simulink subsystem "PvtSubSys_VSM_SCM"  (R2020b)
settings: Solver=VariableStepAuto  StartTime=0.0  StopTime=10.0  RelTol=1e-3
undefined symbols (not defined in the file): P_Global_VehicleWidthMin_m, P_VSM_LDW_State_Param_LaneTime, P_VSM_LDW_State_Param_Speed, P_VSM_LKA_State_Param_Offset, P_VSM_LSMC_SampleTime
libraries: simulink x45
(part 2 of 3)

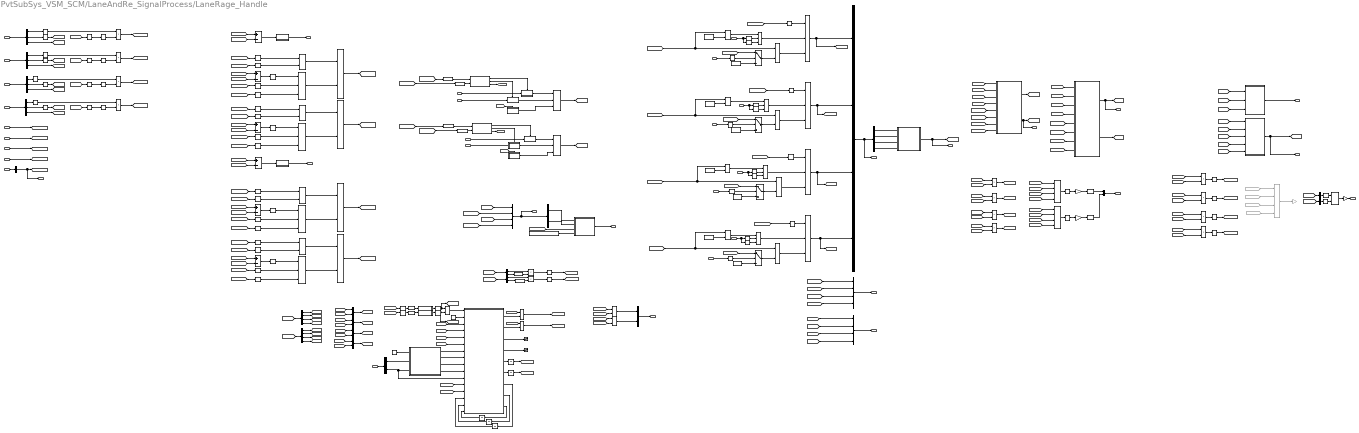
== system PvtSubSys_VSM_SCM/LaneAndRe_SignalProcess/LaneRage_Handle ==
  note: 该目标为相关侧有效
      | 车道线
  note: 注意：由于后期模块没有使用该
      | 输出（lane1）；所以去掉该输出
      | 接口；
      | 2020/10/12
  note: 目标车道线输出；
      | T_Valid为bool；
      | 其余皆为Single；
  note: 去掉了输出L信号；
      | 因为后面模块用不到；
  note: 车道线与车道边界之间差值（0.3m）；
  note: 存在数据类型问题：bool*double，需要求改
  Left_Lane : Inport
  Right_Lane : Inport  Port=2
  Left_Re : Inport  Port=3
  Right_Re : Inport  Port=4
  L_Lvalid : Inport  Port=5
  R_Lvalid : Inport  Port=6
  L_Revalid : Inport  Port=7
  R_Revalid : Inport  Port=8
  Center_lane : Inport  Port=9
  EVI : Inport  Port=10
  PilotSts : Inport  Port=11
  Abs{,1..13} (14 alike) : Abs
  Add{1..6} (6 alike) : Sum  Inputs=+-
  Atan : Trigonometry  Operator=atan
  Atan1 : Trigonometry  Operator=atan
  Bus Creator{,2,4,9} (4 alike) : BusCreator  Inputs=4
  Bus Creator{1,3,5..8} (6 alike) : BusCreator  Inputs=2
  Bus Selector : BusSelector  OutputSignals=Left_LaneValid,Right_LaneValid,Left_ReValid,Right_ReValid
  Bus Selector{1..4} (4 alike) : BusSelector  OutputSignals=A0,A1,A2
  Bus Selector10 : BusSelector  OutputSignals=A2
  Bus Selector11 : BusSelector  OutputSignals=A0,A1,A2,A3
  Bus Selector12 : BusSelector  OutputSignals=A0,A1,A2,A3
  Bus Selector13 : BusSelector  OutputSignals=Kap,VehicleSpd_ms
  Bus Selector5 : BusSelector  OutputSignals=A0,Valid
  Bus Selector6 : BusSelector  OutputSignals=A0,Valid
  Bus Selector7 : BusSelector  OutputSignals=Left_ValidLane,Right_ValidLane
  Bus Selector8 : BusSelector  OutputSignals=lane_Center
  Bus Selector9 : BusSelector  OutputSignals=A2
  CalcEgoVehMove1 : MATLAB Function  TreatAsAtomicUnit=on
  Compare To Constant{,23,37..38} (4 alike) : simulink/Logic and Bit Operations/Compare To Constant  relop=<  const=0.5  OutDataTypeStr=boolean
  Compare To Constant24 : simulink/Logic and Bit Operations/Compare To Constant  relop=>  const=4  OutDataTypeStr=boolean
  Compare To Constant25 : simulink/Logic and Bit Operations/Compare To Constant  relop=<  const=0  OutDataTypeStr=boolean
  Compare To Constant26 : simulink/Logic and Bit Operations/Compare To Constant  relop=>  const=0  OutDataTypeStr=boolean
  Compare To Constant34 : simulink/Logic and Bit Operations/Compare To Constant  relop=<  const=3.5  OutDataTypeStr=boolean
  Compare To Constant39 : simulink/Logic and Bit Operations/Compare To Constant  relop=>  const=0  OutDataTypeStr=boolean
  Compare To Constant40 : simulink/Logic and Bit Operations/Compare To Constant  relop=>  const=0  OutDataTypeStr=boolean
  Compare To Constant41 : simulink/Logic and Bit Operations/Compare To Constant  relop=>  const=0.2  OutDataTypeStr=boolean
  Compare To Constant42 : simulink/Logic and Bit Operations/Compare To Constant  relop=>  const=0.2  OutDataTypeStr=boolean
  Compare To Constant{47,49,51,53} (4 alike) : simulink/Logic and Bit Operations/Compare To Constant  relop===  const=2  OutDataTypeStr=boolean
  Compare To Constant{48,50,52,54} (4 alike) : simulink/Logic and Bit Operations/Compare To Constant  relop===  const=3  OutDataTypeStr=boolean
  Compare To Zero{,1,4..5,7..8,10..14,16..20,22..25,28..29} (22 alike) : simulink/Logic and Bit Operations/Compare To Zero  relop=>  OutDataTypeStr=boolean
  Compare To Zero2 : simulink/Logic and Bit Operations/Compare To Zero  relop=<  OutDataTypeStr=boolean
  Compare To Zero26 : simulink/Logic and Bit Operations/Compare To Zero  relop=<  OutDataTypeStr=boolean
  Constant1 : Constant  Value=[1,1]  OutDataTypeStr=uint8
  Constant{5,7,10,14} (4 alike) : Constant  Value=single(998)
  Constant{3,11,13,15} (4 alike) : Constant  Value=single(2.75)
  Constant12 : Constant  Value=0.02  OutDataTypeStr=single
  Constant9 : Constant  Value=P_VSM_LKA_State_Param_Offset
  Cos{,1..3} (4 alike) : Trigonometry  Operator=cos
  Data Type Conversion{,5..7,9..10} (6 alike) : DataTypeConversion
  Data Type Conversion2 : DataTypeConversion  OutDataTypeStr=double
  Data Type Conversion4 : DataTypeConversion  OutDataTypeStr=double
  Divide{,1..12,15} (14 alike) : Product  Inputs=**
  ELK_laneValid : MATLAB Function  TreatAsAtomicUnit=on
  From87 : From  Commented=on  GotoTag=Left_LaneA2
  From88 : From  Commented=on  GotoTag=Right_LaneA2
  From89 : From  Commented=on  GotoTag=Left_ReA2
  From90 : From  Commented=on  GotoTag=Right_ReA2
  Gain : Gain  Commented=on  Gain=2
  Gain1 : Gain  Gain=2
  Gain2 : Gain  Gain=57.3
  Gain3 : Gain  Gain=57.3
  If : If  NumInputs=2  ElseIfExpressions=u2>0
  If1 : If  NumInputs=2  ElseIfExpressions=u2>0
  L_Lvalid1 : InportShadow  Port=5
  L_Revalid1 : InportShadow  Port=7
  Left_Lane1 : InportShadow
  Left_Re1 : InportShadow  Port=3
  Logical Operator{,25,27,32..33,40..41} (7 alike) : Logic  Operator=OR  AllPortsSameDT=off  OutDataTypeStr=boolean
  Logical Operator{4..7,24,30..31,36} (8 alike) : Logic  Inputs=3  AllPortsSameDT=off  OutDataTypeStr=boolean
  Logical Operator{28..29,34..35,38..39} (6 alike) : Logic  AllPortsSameDT=off  OutDataTypeStr=boolean
  Logical Operator{44..47} (4 alike) : Logic  Operator=OR  Inputs=3  AllPortsSameDT=off  OutDataTypeStr=boolean
  MATLAB Function : MATLAB Function  TreatAsAtomicUnit=on
  MATLAB Function1 : MATLAB Function  TreatAsAtomicUnit=on
  MATLAB Function2 : MATLAB Function  TreatAsAtomicUnit=on
  Max : MinMax  Commented=on  Function=max  Inputs=4
  Max1 : MinMax  Function=max  Inputs=4
  Max2 : MinMax  Function=max  Inputs=4
  Max3 : MinMax  Function=max  Inputs=2
  Merge : Merge  Inputs=3
  Merge1 : Merge  Inputs=3
  PilotSts3 : InportShadow  Port=11
  PilotSts4 : InportShadow  Port=11
  PilotSts5 : InportShadow  Port=11
  R_Lvalid1 : InportShadow  Port=6
  R_Revalid1 : InportShadow  Port=8
  Relational Operator{1..4,9..10,13..14} (8 alike) : RelationalOperator  Operator=<  OutDataTypeStr=boolean  RndMeth=Nearest
  Right_Lane1 : InportShadow  Port=2
  Right_Re1 : InportShadow  Port=4
  SameTwoLaneCondition : MATLAB Function  TreatAsAtomicUnit=on
  SingleLaneCondition : MATLAB Function  TreatAsAtomicUnit=on
  Subsystem : Subsystem
  Subsystem4 : Subsystem  mask{Ts=P_VSM_LSMC_SampleTime, Max=10}
      mask prompts: Ts "Sample Time:"; Max "Max Limit:"
      mask Display:
      | Ts=get_param(gcb,'Ts');
      | Max=get_param(gcb,'Max');
      | disp(['Ts:' Ts '\n' 'Max:' Max ]);
  Subsystem6 : Subsystem  mask{Ts=P_VSM_LSMC_SampleTime, Max=10}
      mask prompts: Ts "Sample Time:"; Max "Max Limit:"
      mask Display:
      | Ts=get_param(gcb,'Ts');
      | Max=get_param(gcb,'Max');
      | disp(['Ts:' Ts '\n' 'Max:' Max ]);
  Switch Case Action Subsystem : Subsystem  TreatAsAtomicUnit=on
  Switch Case Action Subsystem1 : Subsystem  TreatAsAtomicUnit=on
  Switch Case Action Subsystem2 : Subsystem  TreatAsAtomicUnit=on
  Switch Case Action Subsystem3 : Subsystem  TreatAsAtomicUnit=on
  Switch Case Action Subsystem4 : Subsystem  TreatAsAtomicUnit=on
  Switch Case Action Subsystem5 : Subsystem  TreatAsAtomicUnit=on
  Switch{1,3,5,7} (4 alike) : Switch  Criteria=u2 > Threshold
  Terminator : Terminator
  Terminator2 : Terminator
  Tracker : MATLAB Function  TreatAsAtomicUnit=on
  TwoLaneCondition : MATLAB Function  TreatAsAtomicUnit=on
  Unit Delay{2..6} (5 alike) : UnitDelay  SampleTime=-1  HasFrameUpgradeWarning=on
  atan{,1..3} (4 alike) : Trigonometry  Operator=atan
  Left_LaneRe30 : Outport
  Right_LaneRe30 : Outport  Port=2
  LaneValid : Outport  Port=3
  HeadingAngle : Outport  Port=4
  LaneCurve : Outport  Port=5
  Valid_Lane : Outport  Port=6
  LaneChangeValid : Outport  Port=7
  Center_Lane : Outport  Port=8
  LDWLKAELK_LWidth : Outport  Port=9
  LSM_LCK_CLane : Outport  Port=10
  Related_Lane : Outport  Port=11
  LSS_RFMHandel_LaneA0 : Outport  Port=12
  Signal_Lane1 : Outport  Port=13
  Signal_Lane2 : Outport  Port=14
  Signal_Lane3 : Outport  Port=15
  LSS_RFM_LaneA1 : Outport  Port=16
  wires:
  Gain1/1 -> LaneCurve/1
  Max3/1 -> Gain1/1
  Bus Selector10/1 -> Abs12/1  "<A2>"
  Bus Selector9/1 -> Abs13/1  "<A2>"
  [Left_ValidLane] -> Bus Selector9/1
  [Right_ValidLane] -> Bus Selector10/1
  Constant9/1 -> Subsystem/4(Offset)
  [Center_Lane] -> Subsystem/3(CenterLane)
  Bus Selector8/1 -> LSM_LCK_CLane/1, [Center_Lane]  "<lane_Center>"
  Center_lane/1 -> Bus Selector8/1
  Bus Selector7/2 -> Subsystem/2(<Right_ValidLane>)  "<Right_ValidLane>"
  Bus Selector7/1 -> Subsystem/1(<Left_ValidLane>)  "<Left_ValidLane>"
  [Host_RRE] -> Bus Creator2/4  "Host_RRE"
  [Host_LRE] -> Bus Creator2/2  "Host_LRE"
  MATLAB Function2/1(y) -> Right_LaneRe30/1
  [Right_LaneOp_A0] -> Add3/2
  [Right_ReOp_A0] -> Add3/1
  Add3/1 -> MATLAB Function2/1(u)
  MATLAB Function1/1(y) -> Left_LaneRe30/1
  Compare To Zero29/1 -> Logical Operator31/3
  Compare To Zero28/1 -> Logical Operator31/2
  [Orginal_R_Lvalid] -> Compare To Zero28/1
  [Orginal_R_Revalid] -> Compare To Zero29/1
  [Orginal_R_Lvalid] -> Compare To Zero20/1
  Logical Operator31/1 -> Logical Operator32/2
  Compare To Zero20/1 -> Logical Operator35/1
  [Right_ReOp_A0] -> Add5/2
  [Right_LaneOp_A0] -> Add5/1
  Add5/1 -> Compare To Zero26/1
  Compare To Zero26/1 -> Logical Operator31/1
  [Orginal_R_Revalid] -> Compare To Constant23/1
  Compare To Constant23/1 -> Logical Operator35/2
  Logical Operator35/1 -> Logical Operator32/1
  Logical Operator32/1 -> [Host_RLane]
  Logical Operator34/1 -> Logical Operator33/1
  Compare To Zero22/1 -> Logical Operator34/2
  [Orginal_R_Revalid] -> Compare To Zero22/1
  Compare To Constant37/1 -> Logical Operator34/1
  [Orginal_R_Lvalid] -> Compare To Constant37/1
  Compare To Zero23/1 -> Logical Operator36/1
  Add6/1 -> Compare To Zero23/1
  [Right_LaneOp_A0] -> Add6/1
  [Right_ReOp_A0] -> Add6/2
  Logical Operator36/1 -> Logical Operator33/2
  [Orginal_R_Revalid] -> Compare To Zero25/1
  [Orginal_R_Lvalid] -> Compare To Zero24/1
  Compare To Zero24/1 -> Logical Operator36/2
  Compare To Zero25/1 -> Logical Operator36/3
  Logical Operator33/1 -> [Host_RRE]
  [Host_LRE] -> Data Type Conversion5/1
  [Host_LLane] -> Data Type Conversion/1
  Logical Operator27/1 -> [Host_LRE]
  Compare To Zero19/1 -> Logical Operator30/3
  Compare To Zero18/1 -> Logical Operator30/2
  [Orginal_L_Lvalid] -> Compare To Zero18/1
  [Orginal_L_Revalid] -> Compare To Zero19/1
  Logical Operator30/1 -> Logical Operator27/2
  [Left_ReOp_A0] -> Add4/2
  [Left_LaneOp_A0] -> Add4/1
  Add4/1 -> Compare To Zero17/1
  Compare To Zero17/1 -> Logical Operator30/1
  [Orginal_L_Lvalid] -> Compare To Constant/1
  Compare To Constant/1 -> Logical Operator28/1
  [Orginal_L_Revalid] -> Compare To Zero16/1
  Compare To Zero16/1 -> Logical Operator28/2
  Logical Operator28/1 -> Logical Operator27/1
  Logical Operator25/1 -> [Host_LLane]
  Logical Operator29/1 -> Logical Operator25/1
  Compare To Constant38/1 -> Logical Operator29/2
  [Orginal_L_Revalid] -> Compare To Constant38/1
  [Left_LaneOp_A0] -> Add2/2
  [Left_ReOp_A0] -> Add2/1
  Compare To Zero2/1 -> Logical Operator24/1
  Add1/1 -> Compare To Zero2/1
  [Left_LaneOp_A0] -> Add1/1
  [Left_ReOp_A0] -> Add1/2
  Compare To Zero12/1 -> Logical Operator29/1
  Logical Operator24/1 -> Logical Operator25/2
  [Orginal_L_Lvalid] -> Compare To Zero12/1
  [Orginal_L_Revalid] -> Compare To Zero5/1
  [Orginal_L_Lvalid] -> Compare To Zero4/1
  Compare To Zero4/1 -> Logical Operator24/2
  Compare To Zero5/1 -> Logical Operator24/3
  Add2/1 -> MATLAB Function1/1(u)
  Bus Creator3/1 -> LaneChangeValid/1
  Compare To Constant26/1 -> [RightChange_old]  "VSM_RightChange_old"
  Compare To Constant25/1 -> [LeftChange_old]  "VSM_LeftChange_old"
  Switch Case Action Subsystem5/1(Out1) -> Merge1/3
  [Right_else] -> Switch Case Action Subsystem5/Action
  Switch Case Action Subsystem4/1(Out1) -> Merge/3
  [Left_else] -> Switch Case Action Subsystem4/Action
  Divide12/1 -> Compare To Constant26/1
  Divide11/1 -> Compare To Constant25/1
  Bus Selector6/2 -> Data Type Conversion9/1  "<Valid>"
  Bus Selector6/1 -> Divide12/1  "<A0>"
  Bus Selector5/2 -> Data Type Conversion10/1  "<Valid>"
  Bus Selector5/1 -> Divide11/1  "<A0>"
  [Right_ValidLane] -> Bus Selector6/1  "Right_ValidLane"
  [Left_ValidLane] -> Bus Selector5/1  "Left_ValidLane"
  Bus Creator2/1 -> Valid_Lane/1, Bus Selector7/1
  [Right_ValidLane] -> Bus Creator2/3  "Right_ValidLane"
  [Left_ValidLane] -> Bus Creator2/1  "Left_ValidLane"
  Data Type Conversion7/1 -> If1/2
  Data Type Conversion6/1 -> If1/1
  Data Type Conversion5/1 -> If/2
  Data Type Conversion/1 -> If/1
  Merge1/1 -> [Right_ValidLane]
  Merge/1 -> [Left_ValidLane]
  If1/3 -> [Right_else]
  Switch Case Action Subsystem3/1(Out1) -> Merge1/2
  Switch Case Action Subsystem2/1(Out1) -> Merge1/1
  If1/2 -> Switch Case Action Subsystem3/Action
  If1/1 -> Switch Case Action Subsystem2/Action
  Right_Re1/1 -> Switch Case Action Subsystem3/1(In1)  "Right_Re"
  Right_Lane1/1 -> Switch Case Action Subsystem2/1(In1)  "Right_Lane"
  Switch Case Action Subsystem1/1(Out1) -> Merge/2
  Switch Case Action Subsystem/1(Out1) -> Merge/1
  If/3 -> [Left_else]
  [Host_RRE] -> Data Type Conversion7/1
  [Host_RLane] -> Data Type Conversion6/1
  If/2 -> Switch Case Action Subsystem1/Action
  Left_Re1/1 -> Switch Case Action Subsystem1/1(In1)  "Left_Re"
  If/1 -> Switch Case Action Subsystem/Action
  Left_Lane1/1 -> Switch Case Action Subsystem/1(In1)  "Left_Lane"
  From89/1 -> Max/3
  From90/1 -> Max/4
  From88/1 -> Max/2
  From87/1 -> Max/1
  Abs11/1 -> [Right_ReA2]
  Abs10/1 -> [Left_ReA2]
  Abs9/1 -> [Right_LaneA2]
  Abs8/1 -> [Left_LaneA2]
  Divide10/1 -> Abs11/1
  Divide9/1 -> Abs10/1
  [Right_Re_A2] -> Divide10/2
  [Right_ReValid] -> Divide10/1
  [Left_Re_A2] -> Divide9/2
  [Left_ReValid] -> Divide9/1
  [Right_Lane_A2] -> Divide8/2
  [Right_LaneValid] -> Divide8/1
  Bus Selector4/3 -> [Right_Re_A2]  "<A2>"
  Bus Selector3/3 -> [Left_Re_A2]  "<A2>"
  Bus Selector2/3 -> [Right_Lane_A2]  "<A2>"
  Bus Selector1/3 -> [Left_Lane_A2]  "<A2>"
  Bus Selector3/2 -> Abs5/1  "<A1>"
  [Left_LaneValid] -> Divide15/1
  Divide8/1 -> Abs9/1
  [Left_Lane_A2] -> Divide15/2
  Max/1 -> Gain/1
  Divide15/1 -> Abs8/1
  Bus Creator1/1 -> HeadingAngle/1
  [Right_ReA1] -> Max2/4
  [Left_ReA1] -> Max2/3
  [Right_LaneA1] -> Max2/2
  [Left_LaneA1] -> Max2/1
  [Right_ReA1] -> Max1/4
  [Left_ReA1] -> Max1/3
  [Right_LaneA1] -> Max1/2
  [Left_LaneA1] -> Max1/1
  Divide7/1 -> [Right_ReA1]
  Divide6/1 -> [Left_ReA1]
  Divide5/1 -> [Right_LaneA1]
  Divide4/1 -> [Left_LaneA1]
  Compare To Constant24/1 -> Bus Creator1/2  "HeadingAngle_Out"
  Atan1/1 -> Gain3/1
  Max2/1 -> Atan1/1
  [Right_ReValid] -> Divide7/2
  [Right_Re_A1] -> Divide7/1
  [Left_ReValid] -> Divide6/2
  [Left_Re_A1] -> Divide6/1
  [Right_LaneValid] -> Divide5/2
  [Right_Lane_A1] -> Divide5/1
  [Left_LaneValid] -> Divide4/2
  [Left_Lane_A1] -> Divide4/1
  Max1/1 -> Atan/1
  Atan/1 -> Gain2/1
  Compare To Constant34/1 -> Bus Creator1/1  "HeadingAngle_In"
  Abs7/1 -> [Right_Re_A1]
  Abs5/1 -> [Left_Re_A1]
  Abs3/1 -> [Right_Lane_A1]
  Abs1/1 -> [Left_Lane_A1]
  [Right_ReOp_A0] -> SameTwoLaneCondition/8(reright)
  [Left_ReOp_A0] -> SameTwoLaneCondition/7(releft)
  [Right_LaneOp_A0] -> SameTwoLaneCondition/6(laneright)
  [Left_LaneOp_A0] -> SameTwoLaneCondition/5(laneleft)
  Divide3/1 -> [Right_ReOp_A0]
  Divide2/1 -> [Left_ReOp_A0]
  Divide1/1 -> [Right_LaneOp_A0]
  Divide/1 -> [Left_LaneOp_A0]
  Cos3/1 -> Divide3/2
  atan3/1 -> Cos3/1
  [Right_Re_A1] -> atan3/1
  Abs6/1 -> Divide3/1
  Cos2/1 -> Divide2/2
  atan2/1 -> Cos2/1
  [Left_Re_A1] -> atan2/1
  Abs4/1 -> Divide2/1
  atan1/1 -> Cos1/1
  Cos1/1 -> Divide1/2
  [Right_Lane_A1] -> atan1/1
  Abs2/1 -> Divide1/1
  Abs/1 -> Divide/1
  Cos/1 -> Divide/2
  atan/1 -> Cos/1
  [Left_Lane_A1] -> atan/1
  Bus Selector4/2 -> Abs7/1  "<A1>"
  Bus Selector4/1 -> Abs6/1  "<A0>"
  Bus Selector3/1 -> Abs4/1  "<A0>"
  Bus Selector2/1 -> Abs2/1  "<A0>"
  Bus Selector2/2 -> Abs3/1  "<A1>"
  Bus Selector1/2 -> Abs1/1  "<A1>"
  Bus Selector1/1 -> Abs/1  "<A0>"
  Right_Re/1 -> Bus Selector4/1  "Right_Re"
  Left_Re/1 -> Bus Selector3/1  "Left_Re"
  Right_Lane/1 -> Bus Selector2/1  "Right_Lane"
  Left_Lane/1 -> Bus Selector1/1  "Left_Lane"
  MATLAB Function/1(L) -> LDWLKAELK_LWidth/1, [L]  "VSM_ELK_LWidth"
  [lane1] -> MATLAB Function/1(lane1)
  [lane3] -> MATLAB Function/3(lane3)
  [lane2] -> MATLAB Function/2(lane2)
  [L2] -> MATLAB Function/5(L2)
  [L1] -> MATLAB Function/4(L1)
  [lane3] -> ELK_laneValid/3(lane3)
  SameTwoLaneCondition/1(L1) -> [L1]
  Logical Operator4/1 -> [Left_ReValid], Bus Creator/3  "Left_ReValid"
  Logical Operator7/1 -> [Right_ReValid], Bus Creator/4  "Right_ReValid"
  [Left_ReValid] -> TwoLaneCondition/3(releft_valid)
  [Right_ReValid] -> TwoLaneCondition/4(reright_valid)
  [Left_LaneOp_A0] -> TwoLaneCondition/5(laneleft)  "Left_Lane"
  [Right_LaneOp_A0] -> TwoLaneCondition/6(laneright)  "Right_Lane"
  [Left_ReOp_A0] -> TwoLaneCondition/7(releft)  "Left_Re"
  [Right_ReOp_A0] -> TwoLaneCondition/8(reright)  "Right_Re"
  SingleLaneCondition/1(lane) -> Signal_Lane1/1, [lane1]  "lane1"
  SameTwoLaneCondition/2(lane) -> Signal_Lane2/1, [lane2]
  TwoLaneCondition/1(lane) -> Signal_Lane3/1, [lane3]
  Bus Creator/1 -> Related_Lane/1, Bus Selector/1
  [lane1] -> ELK_laneValid/1(lane1)
  [lane2] -> ELK_laneValid/2(lane2)
  ELK_laneValid/1(y) -> LaneValid/1
  TwoLaneCondition/2(L2) -> [L2]
  Logical Operator6/1 -> [Right_LaneValid], Bus Creator/2  "Right_LaneValid"
  Logical Operator5/1 -> [Left_LaneValid], Bus Creator/1  "Left_LaneValid"
  Compare To Zero/1 -> Logical Operator5/1
  Relational Operator9/1 -> Logical Operator5/3
  [Left_LaneOp_A0] -> Relational Operator1/1, Relational Operator9/1  "Left_Lane"
  [Left_LaneValid] -> TwoLaneCondition/1(laneleft_valid)
  [Right_LaneValid] -> TwoLaneCondition/2(laneright_valid)
  [Left_ReOp_A0] -> Switch1/1  "Left_Re"
  Switch1/1 -> Relational Operator9/2
  Constant14/1 -> Switch1/3
  Compare To Zero7/1 -> Switch1/2
  L_Revalid1/1 -> Compare To Zero7/1
  R_Revalid1/1 -> Compare To Zero10/1
  Compare To Zero10/1 -> Switch3/2
  Constant5/1 -> Switch3/3
  Switch3/1 -> Relational Operator13/2
  [Right_ReOp_A0] -> Switch3/1  "Right_Re"
  [Right_LaneOp_A0] -> Relational Operator2/1, Relational Operator13/1  "Right_Lane"
  Relational Operator13/1 -> Logical Operator6/3
  Compare To Zero8/1 -> Logical Operator6/1
  Compare To Zero11/1 -> Logical Operator4/1
  Relational Operator10/1 -> Logical Operator4/3
  [Left_ReOp_A0] -> Relational Operator3/1, Relational Operator10/1  "Left_Re"
  [Left_LaneOp_A0] -> Switch5/1  "Left_Lane"
  Switch5/1 -> Relational Operator10/2
  Constant10/1 -> Switch5/3
  Compare To Zero1/1 -> Switch5/2
  L_Lvalid1/1 -> Compare To Zero1/1
  R_Lvalid1/1 -> Compare To Zero13/1
  Compare To Zero13/1 -> Switch7/2
  Constant7/1 -> Switch7/3
  Switch7/1 -> Relational Operator14/2
  [Right_LaneOp_A0] -> Switch7/1  "Right_Lane"
  [Right_ReOp_A0] -> Relational Operator4/1, Relational Operator14/1  "Right_Re"
  Relational Operator14/1 -> Logical Operator7/3
  Compare To Zero14/1 -> Logical Operator7/1
  Constant13/1 -> Relational Operator1/2
  Constant3/1 -> Relational Operator2/2
  Constant11/1 -> Relational Operator3/2
  Constant15/1 -> Relational Operator4/2
  Bus Selector/1 -> SingleLaneCondition/1(laneleft_valid)  "<Left_LaneValid>"
  Bus Selector/2 -> SingleLaneCondition/2(laneright_valid)  "<Right_LaneValid>"
  Bus Selector/3 -> SingleLaneCondition/3(releft_valid)  "<Left_ReValid>"
  Bus Selector/4 -> SingleLaneCondition/4(reright_valid)  "<Right_ReValid>"
  [Left_LaneValid] -> SameTwoLaneCondition/1(laneleft_valid)
  [Right_LaneValid] -> SameTwoLaneCondition/2(laneright_valid)
  [Left_ReValid] -> SameTwoLaneCondition/3(releft_valid)
  [Right_ReValid] -> SameTwoLaneCondition/4(reright_valid)
  L_Lvalid/1 -> [Orginal_L_Lvalid]
  R_Lvalid/1 -> [Orginal_R_Lvalid]
  L_Revalid/1 -> [Orginal_L_Revalid]
  R_Revalid/1 -> [Orginal_R_Revalid]
  [Orginal_L_Lvalid] -> Compare To Zero/1
  [Orginal_R_Lvalid] -> Compare To Zero8/1
  [Orginal_L_Revalid] -> Compare To Zero11/1
  [Orginal_R_Revalid] -> Compare To Zero14/1
  Subsystem/1(Out1) -> Center_Lane/1
  Data Type Conversion9/1 -> Divide12/2
  Data Type Conversion10/1 -> Divide11/2
  Gain2/1 -> Compare To Constant34/1
  Gain3/1 -> Compare To Constant24/1
  Abs12/1 -> Max3/2
  Abs13/1 -> Max3/1
  [Right_LaneValid] -> Compare To Constant40/1
  [A1] -> Tracker/4(A1)
  Bus Selector11/3 -> [LA2]  "<A2>"
  Bus Creator8/1 -> [A3]
  Logical Operator41/1 -> Bus Creator3/2  "RightChange"
  [RightChange_old] -> Logical Operator41/1
  Tracker/7(pre_A1_1) -> Unit Delay6/1
  Bus Creator5/1 -> [A0]
  Logical Operator40/1 -> Bus Creator3/1  "LeftChange"
  [LValid] -> Logical Operator38/1
  [RightChange_new] -> Logical Operator41/2
  Data Type Conversion2/1 -> Subsystem4/1(In1)
  Compare To Constant41/1 -> [RValid], Logical Operator/2
  Tracker/3(error_right) -> Terminator2/1  "VSM_ERROR_RIGHT"
  [LeftChange_new] -> Logical Operator40/2
  Compare To Constant39/1 -> Data Type Conversion4/1
  [RA2] -> Bus Creator7/1
  [LeftChange_old] -> Logical Operator40/1
  Bus Selector12/2 -> [RA1]  "<A1>"
  Bus Selector12/1 -> [RA0]  "<A0>"
  [pre_A1_2K1] -> Tracker/12(pre_A1_2K1)
  Compare To Constant42/1 -> [LValid], Logical Operator/1
  Bus Selector11/2 -> [LA1]  "<A1>"
  Bus Selector11/1 -> [LA0]  "<A0>"
  [RValid] -> Logical Operator39/1
  Subsystem4/1(Out1) -> Compare To Constant41/1
  Tracker/2(RightOffset_b) -> Logical Operator39/2
  CalcEgoVehMove1/4(SinOfPsi) -> Tracker/10(SinOfPsi)
  Unit Delay2/1 -> [pre_A1_2K1]
  [pre_A0_2K1] -> Tracker/13(pre_A0_2K1)
  Tracker/1(LeftOffset_b) -> Logical Operator38/2
  Logical Operator38/1 -> [LeftChange_new]  "VSM_LeftChange_new"
  Unit Delay3/1 -> [pre_A0_2K1]
  Bus Creator6/1 -> [A1]
  Tracker/5(pre_A1_2) -> Unit Delay2/1
  Logical Operator39/1 -> [RightChange_new]  "VSM_RightChange_new"
  Bus Selector13/2 -> CalcEgoVehMove1/3(Vego), Tracker/11(vRef)  "<VehicleSpd_ms>"
  CalcEgoVehMove1/3(CosOfPsi) -> Tracker/9(CosOfPsi)
  Unit Delay6/1 -> Tracker/14(pre_A1_1K1)
  Tracker/8(pre_A0_1) -> Unit Delay5/1
  Unit Delay4/1 -> Tracker/16(pre_LineConfK1)
  Bus Selector13/1 -> CalcEgoVehMove1/2(Kap)  "<Kap>"
  [Left_ValidLane] -> Bus Selector11/1
  [Left_LaneValid] -> Compare To Constant39/1
  Data Type Conversion4/1 -> Subsystem6/1(In1)
  EVI/1 -> Bus Selector13/1
  Subsystem6/1(Out1) -> Compare To Constant42/1
  Tracker/9(pre_LineConf) -> Unit Delay4/1
  Compare To Constant40/1 -> Data Type Conversion2/1
  [LA2] -> Bus Creator7/2
  Constant1/1 -> Tracker/2(LineConf)
  [LA3] -> Bus Creator8/2
  Constant12/1 -> CalcEgoVehMove1/1(tCycle)
  [A0] -> Tracker/3(A0)
  [A2] -> Tracker/5(A2)
  [RA3] -> Bus Creator8/1
  Unit Delay5/1 -> Tracker/15(pre_A0_1K1)
  [A3] -> Tracker/6(A3)
  Bus Creator7/1 -> [A2]
  [LA1] -> Bus Creator6/2
  Bus Selector11/4 -> [LA3]  "<A3>"
  [RA1] -> Bus Creator6/1
  Logical Operator/1 -> Tracker/1(LineUpdate)
  Bus Selector12/4 -> [RA3]  "<A3>"
  CalcEgoVehMove1/1(dDeltaX) -> Tracker/7(dDeltaX)
  [Right_ValidLane] -> Bus Selector12/1
  Tracker/4(error_left) -> Terminator/1  "VSM_ERROR_LEFT"
  [LA0] -> Bus Creator5/2
  Tracker/6(pre_A0_2) -> Unit Delay3/1
  [RA0] -> Bus Creator5/1
  CalcEgoVehMove1/2(dDeltaY) -> Tracker/8(dDeltaY)
  Bus Selector12/3 -> [RA2]  "<A2>"
  Compare To Constant47/1 -> Logical Operator44/2
  Compare To Constant48/1 -> Logical Operator44/3
  PilotSts/1 -> Compare To Constant47/1, Compare To Constant48/1
  Relational Operator1/1 -> Logical Operator44/1
  Logical Operator44/1 -> Logical Operator5/2
  PilotSts3/1 -> Compare To Constant50/1, Compare To Constant49/1
  Compare To Constant50/1 -> Logical Operator45/3
  Compare To Constant49/1 -> Logical Operator45/2
  Relational Operator2/1 -> Logical Operator45/1
  Logical Operator45/1 -> Logical Operator6/2
  Compare To Constant51/1 -> Logical Operator46/2
  Compare To Constant52/1 -> Logical Operator46/3
  PilotSts4/1 -> Compare To Constant51/1, Compare To Constant52/1
  Relational Operator3/1 -> Logical Operator46/1
  Logical Operator46/1 -> Logical Operator4/2
  PilotSts5/1 -> Compare To Constant54/1, Compare To Constant53/1
  Compare To Constant54/1 -> Logical Operator47/3
  Compare To Constant53/1 -> Logical Operator47/2
  Relational Operator4/1 -> Logical Operator47/1
  Logical Operator47/1 -> Logical Operator7/2
  [Left_LaneOp_A0] -> Bus Creator4/1  "Left_LaneOp_A0"
  [Right_LaneOp_A0] -> Bus Creator4/2  "Right_LaneOp_A0"
  [Left_ReOp_A0] -> Bus Creator4/3  "Left_ReOp_A0"
  [Right_ReOp_A0] -> Bus Creator4/4  "Right_ReOp_A0"
  Bus Creator4/1 -> LSS_RFMHandel_LaneA0/1
  [Left_Lane_A1] -> Bus Creator9/1  "Left_Lane_A1"
  [Right_Lane_A1] -> Bus Creator9/2  "Right_Lane_A1"
  [Left_Re_A1] -> Bus Creator9/3  "Left_Re_A1"
  [Right_Re_A1] -> Bus Creator9/4  "Right_Re_A1"
  Bus Creator9/1 -> LSS_RFM_LaneA1/1

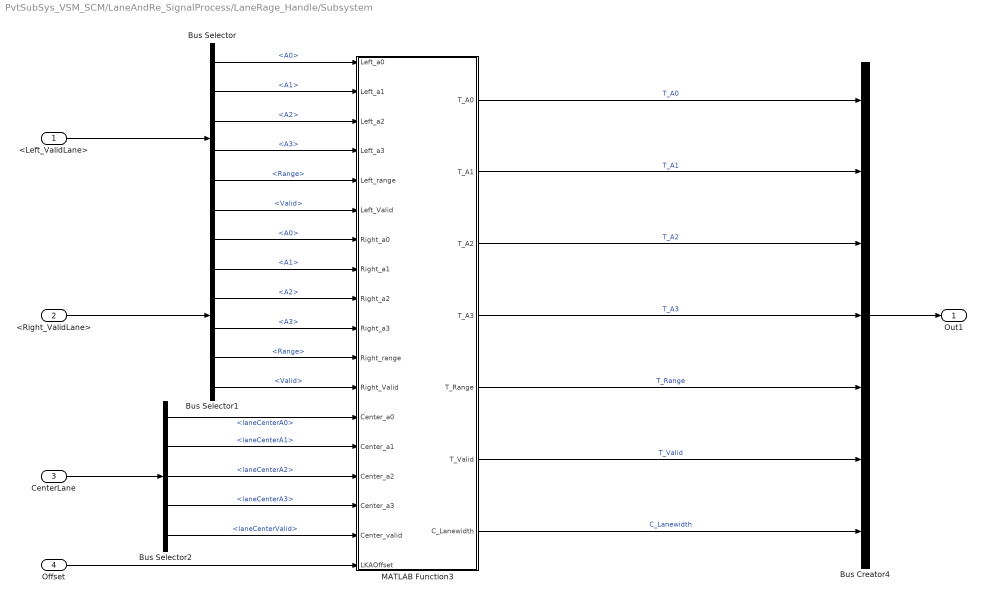
== system PvtSubSys_VSM_SCM/LaneAndRe_SignalProcess/LaneRage_Handle/Subsystem ==
  <Left_ValidLane> : Inport
  <Right_ValidLane> : Inport  Port=2
  CenterLane : Inport  Port=3
  Offset : Inport  Port=4
  Bus Creator4 : BusCreator  Inputs=7
  Bus Selector : BusSelector  OutputSignals=A0,A1,A2,A3,Range,Valid
  Bus Selector1 : BusSelector  OutputSignals=A0,A1,A2,A3,Range,Valid
  Bus Selector2 : BusSelector  OutputSignals=laneCenterA0,laneCenterA1,laneCenterA2,laneCenterA3,laneCenterValid
  MATLAB Function3 : MATLAB Function  TreatAsAtomicUnit=on
  Out1 : Outport
  wires:
  MATLAB Function3/1(T_A0) -> Bus Creator4/1  "T_A0"
  MATLAB Function3/5(T_Range) -> Bus Creator4/5  "T_Range"
  MATLAB Function3/3(T_A2) -> Bus Creator4/3  "T_A2"
  MATLAB Function3/2(T_A1) -> Bus Creator4/2  "T_A1"
  MATLAB Function3/7(C_Lanewidth) -> Bus Creator4/7  "C_Lanewidth"
  MATLAB Function3/4(T_A3) -> Bus Creator4/4  "T_A3"
  MATLAB Function3/6(T_Valid) -> Bus Creator4/6  "T_Valid"
  Offset/1 -> MATLAB Function3/18(LKAOffset)
  Bus Creator4/1 -> Out1/1
  <Left_ValidLane>/1 -> Bus Selector/1
  <Right_ValidLane>/1 -> Bus Selector1/1
  CenterLane/1 -> Bus Selector2/1
  Bus Selector/1 -> MATLAB Function3/1(Left_a0)  "<A0>"
  Bus Selector/2 -> MATLAB Function3/2(Left_a1)  "<A1>"
  Bus Selector/3 -> MATLAB Function3/3(Left_a2)  "<A2>"
  Bus Selector/4 -> MATLAB Function3/4(Left_a3)  "<A3>"
  Bus Selector/5 -> MATLAB Function3/5(Left_range)  "<Range>"
  Bus Selector/6 -> MATLAB Function3/6(Left_Valid)  "<Valid>"
  Bus Selector1/1 -> MATLAB Function3/7(Right_a0)  "<A0>"
  Bus Selector1/2 -> MATLAB Function3/8(Right_a1)  "<A1>"
  Bus Selector1/3 -> MATLAB Function3/9(Right_a2)  "<A2>"
  Bus Selector1/4 -> MATLAB Function3/10(Right_a3)  "<A3>"
  Bus Selector1/5 -> MATLAB Function3/11(Right_range)  "<Range>"
  Bus Selector1/6 -> MATLAB Function3/12(Right_Valid)  "<Valid>"
  Bus Selector2/1 -> MATLAB Function3/13(Center_a0)  "<laneCenterA0>"
  Bus Selector2/2 -> MATLAB Function3/14(Center_a1)  "<laneCenterA1>"
  Bus Selector2/3 -> MATLAB Function3/15(Center_a2)  "<laneCenterA2>"
  Bus Selector2/4 -> MATLAB Function3/16(Center_a3)  "<laneCenterA3>"
  Bus Selector2/5 -> MATLAB Function3/17(Center_valid)  "<laneCenterValid>"

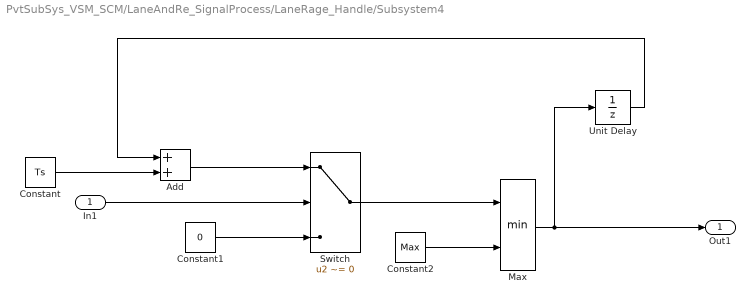
== system PvtSubSys_VSM_SCM/LaneAndRe_SignalProcess/LaneRage_Handle/Subsystem4 ==
  In1 : Inport
  Add : Sum
  Constant : Constant  Value=Ts
  Constant1 : Constant  Value=0
  Constant2 : Constant  Value=Max
  Max : MinMax  Inputs=2
  Switch : Switch  Criteria=u2 ~= 0
  Unit Delay : UnitDelay  SampleTime=-1  HasFrameUpgradeWarning=on
  Out1 : Outport
  wires:
  Switch/1 -> Max/1
  Constant2/1 -> Max/2
  Max/1 -> Out1/1, Unit Delay/1
  Add/1 -> Switch/1
  Constant1/1 -> Switch/3
  Constant/1 -> Add/2
  In1/1 -> Switch/2
  Unit Delay/1 -> Add/1

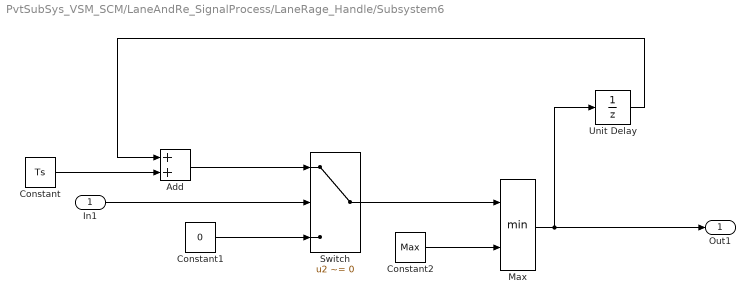
== system PvtSubSys_VSM_SCM/LaneAndRe_SignalProcess/LaneRage_Handle/Subsystem6 ==
  In1 : Inport
  Add : Sum
  Constant : Constant  Value=Ts
  Constant1 : Constant  Value=0
  Constant2 : Constant  Value=Max
  Max : MinMax  Inputs=2
  Switch : Switch  Criteria=u2 ~= 0
  Unit Delay : UnitDelay  SampleTime=-1  HasFrameUpgradeWarning=on
  Out1 : Outport
  wires:
  Unit Delay/1 -> Add/1
  In1/1 -> Switch/2
  Constant/1 -> Add/2
  Constant1/1 -> Switch/3
  Add/1 -> Switch/1
  Max/1 -> Unit Delay/1, Out1/1
  Constant2/1 -> Max/2
  Switch/1 -> Max/1

== system PvtSubSys_VSM_SCM/LaneAndRe_SignalProcess/LaneRage_Handle/Switch Case Action Subsystem ==
  In1 : Inport
  Action Port : ActionPort
  Bus Creator : BusCreator  Inputs=7
  Bus Selector : BusSelector  OutputSignals=A0,A1,A2,A3,Range,Valid,Left_Type
  Out1 : Outport
  wires:
  Bus Selector/7 -> Bus Creator/7  "<Left_Type>"
  Bus Creator/1 -> Out1/1
  Bus Selector/5 -> Bus Creator/5  "<Range>"
  Bus Selector/1 -> Bus Creator/1  "<A0>"
  Bus Selector/6 -> Bus Creator/6  "<Valid>"
  Bus Selector/2 -> Bus Creator/2  "<A1>"
  Bus Selector/4 -> Bus Creator/4  "<A3>"
  Bus Selector/3 -> Bus Creator/3  "<A2>"
  In1/1 -> Bus Selector/1

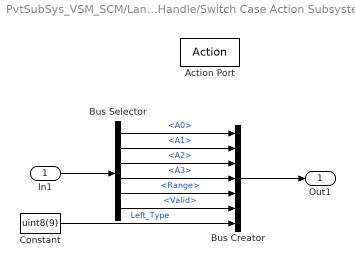
== system PvtSubSys_VSM_SCM/LaneAndRe_SignalProcess/LaneRage_Handle/Switch Case Action Subsystem1 ==
  In1 : Inport
  Action Port : ActionPort
  Bus Creator : BusCreator  Inputs=7
  Bus Selector : BusSelector  OutputSignals=A0,A1,A2,A3,Range,Valid
  Constant : Constant  Value=uint8(9)
  Out1 : Outport
  wires:
  Constant/1 -> Bus Creator/7  "Left_Type"
  In1/1 -> Bus Selector/1
  Bus Selector/3 -> Bus Creator/3  "<A2>"
  Bus Selector/4 -> Bus Creator/4  "<A3>"
  Bus Selector/2 -> Bus Creator/2  "<A1>"
  Bus Selector/6 -> Bus Creator/6  "<Valid>"
  Bus Selector/1 -> Bus Creator/1  "<A0>"
  Bus Selector/5 -> Bus Creator/5  "<Range>"
  Bus Creator/1 -> Out1/1

== system PvtSubSys_VSM_SCM/LaneAndRe_SignalProcess/LaneRage_Handle/Switch Case Action Subsystem2 ==
  In1 : Inport
  Action Port : ActionPort
  Bus Creator : BusCreator  Inputs=7
  Bus Selector : BusSelector  OutputSignals=A0,A1,A2,A3,Range,Valid,Right_Type
  Out1 : Outport
  wires:
  Bus Selector/7 -> Bus Creator/7  "<Right_Type>"
  Bus Creator/1 -> Out1/1
  Bus Selector/5 -> Bus Creator/5  "<Range>"
  Bus Selector/1 -> Bus Creator/1  "<A0>"
  Bus Selector/6 -> Bus Creator/6  "<Valid>"
  Bus Selector/2 -> Bus Creator/2  "<A1>"
  Bus Selector/4 -> Bus Creator/4  "<A3>"
  Bus Selector/3 -> Bus Creator/3  "<A2>"
  In1/1 -> Bus Selector/1

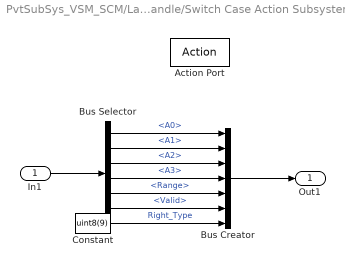
== system PvtSubSys_VSM_SCM/LaneAndRe_SignalProcess/LaneRage_Handle/Switch Case Action Subsystem3 ==
  In1 : Inport
  Action Port : ActionPort
  Bus Creator : BusCreator  Inputs=7
  Bus Selector : BusSelector  OutputSignals=A0,A1,A2,A3,Range,Valid
  Constant : Constant  Value=uint8(9)
  Out1 : Outport
  wires:
  Constant/1 -> Bus Creator/7  "Right_Type"
  In1/1 -> Bus Selector/1
  Bus Selector/3 -> Bus Creator/3  "<A2>"
  Bus Selector/4 -> Bus Creator/4  "<A3>"
  Bus Selector/2 -> Bus Creator/2  "<A1>"
  Bus Selector/6 -> Bus Creator/6  "<Valid>"
  Bus Selector/1 -> Bus Creator/1  "<A0>"
  Bus Selector/5 -> Bus Creator/5  "<Range>"
  Bus Creator/1 -> Out1/1

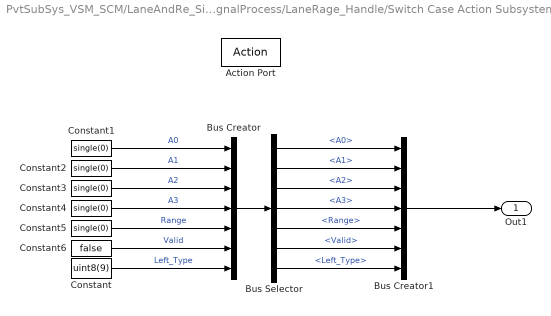
== system PvtSubSys_VSM_SCM/LaneAndRe_SignalProcess/LaneRage_Handle/Switch Case Action Subsystem4 ==
  Action Port : ActionPort
  Bus Creator : BusCreator  Inputs=7
  Bus Creator1 : BusCreator  Inputs=7
  Bus Selector : BusSelector  OutputSignals=A0,A1,A2,A3,Range,Valid,Left_Type
  Constant : Constant  Value=uint8(9)
  Constant{1..5} (5 alike) : Constant  Value=single(0)
  Constant6 : Constant  Value=false
  Out1 : Outport
  wires:
  Bus Creator1/1 -> Out1/1
  Constant5/1 -> Bus Creator/5  "Range"
  Constant1/1 -> Bus Creator/1  "A0"
  Constant6/1 -> Bus Creator/6  "Valid"
  Constant2/1 -> Bus Creator/2  "A1"
  Constant4/1 -> Bus Creator/4  "A3"
  Constant3/1 -> Bus Creator/3  "A2"
  Constant/1 -> Bus Creator/7  "Left_Type"
  Bus Creator/1 -> Bus Selector/1
  Bus Selector/1 -> Bus Creator1/1  "<A0>"
  Bus Selector/2 -> Bus Creator1/2  "<A1>"
  Bus Selector/3 -> Bus Creator1/3  "<A2>"
  Bus Selector/4 -> Bus Creator1/4  "<A3>"
  Bus Selector/5 -> Bus Creator1/5  "<Range>"
  Bus Selector/6 -> Bus Creator1/6  "<Valid>"
  Bus Selector/7 -> Bus Creator1/7  "<Left_Type>"

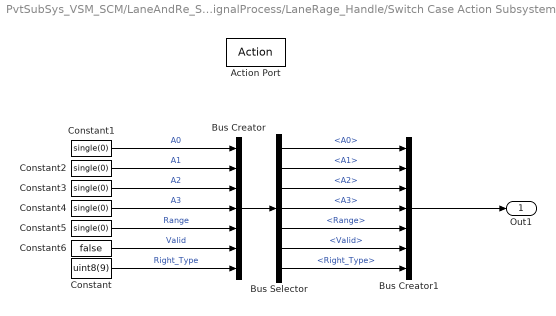
== system PvtSubSys_VSM_SCM/LaneAndRe_SignalProcess/LaneRage_Handle/Switch Case Action Subsystem5 ==
  Action Port : ActionPort
  Bus Creator : BusCreator  Inputs=7
  Bus Creator1 : BusCreator  Inputs=7
  Bus Selector : BusSelector  OutputSignals=A0,A1,A2,A3,Range,Valid,Right_Type
  Constant : Constant  Value=uint8(9)
  Constant{1..5} (5 alike) : Constant  Value=single(0)
  Constant6 : Constant  Value=false
  Out1 : Outport
  wires:
  Bus Selector/7 -> Bus Creator1/7  "<Right_Type>"
  Bus Selector/6 -> Bus Creator1/6  "<Valid>"
  Bus Selector/5 -> Bus Creator1/5  "<Range>"
  Bus Selector/4 -> Bus Creator1/4  "<A3>"
  Bus Selector/3 -> Bus Creator1/3  "<A2>"
  Bus Selector/2 -> Bus Creator1/2  "<A1>"
  Bus Selector/1 -> Bus Creator1/1  "<A0>"
  Bus Creator/1 -> Bus Selector/1
  Constant/1 -> Bus Creator/7  "Right_Type"
  Constant3/1 -> Bus Creator/3  "A2"
  Constant4/1 -> Bus Creator/4  "A3"
  Constant2/1 -> Bus Creator/2  "A1"
  Constant6/1 -> Bus Creator/6  "Valid"
  Constant1/1 -> Bus Creator/1  "A0"
  Constant5/1 -> Bus Creator/5  "Range"
  Bus Creator1/1 -> Out1/1

== matlab function PvtSubSys_VSM_SCM/LKA_LDW_SignalProcess/MATLAB Function ==
  data: FLWhelDy input; FRWhelDy input; preLDY input; LaneCurve input; preFLWhelDy output single; preRDY input; preFRWhelDy output single
function [preFLWhelDy,preFRWhelDy] = fcn(FLWhelDy, FRWhelDy, preLDY, LaneCurve, preRDY)
if LaneCurve>=0.0005
    preFLWhelDy=FLWhelDy;
    preFRWhelDy=FRWhelDy;
else
    preFLWhelDy=preLDY;
    preFRWhelDy=preRDY; 
end

== matlab function PvtSubSys_VSM_SCM/LaneAndRe_SignalProcess/InCondition1/CalcEgoVehMove ==
  data: dDeltaX output single size=1; tCycle input single size=1; Kap input single size=1; Vego input single size=1; alpSideSlipAngle input single size=1; dDeltaY output single size=1; CosOfPsi output single size=1; SinOfPsi output single size=1
function [dDeltaX,dDeltaY,CosOfPsi,SinOfPsi] = EgoVehicleMovement(tCycle,Kap,Vego,alpSideSlipAngle)
%#codegen
if Kap<0.1
    dDeltaX = Vego*tCycle;
    dDeltaY = single(0);
    CosOfPsi = single(1);
    SinOfPsi = single(0);
else
    t_Psi = asin(Kap*Vego*tCycle);
    SinOfPsi = sin(t_Psi);
    CosOfPsi = cos(t_Psi);
    t_dDeltaXTemp = SinOfPsi/Kap;
    t_dDeltaYTemp = single(2*(sin(t_Psi/2)*sin(t_Psi/2))/Kap);
    dDeltaX = cos(alpSideSlipAngle)*t_dDeltaXTemp - sin(alpSideSlipAngle)*t_dDeltaYTemp;
    dDeltaY = sin(alpSideSlipAngle)*t_dDeltaXTemp + cos(alpSideSlipAngle)*t_dDeltaYTemp;
end

== matlab function PvtSubSys_VSM_SCM/LaneAndRe_SignalProcess/InCondition1/MATLAB Function ==
  data: LeftLane output single; A3 input; A2 input; A1 input; A0 input; Range input; RightLane output single; LeftRe output single; RightRe output single
function [LeftLane,RightLane,LeftRe,RightRe] = fcn(A3,A2,A1,A0,Range)
LeftLane=single(zeros(5,1));
RightLane=single(zeros(5,1));
LeftRe=single(zeros(5,1));
RightRe=single(zeros(5,1));
%% leftlane

LeftLane(1)=A3(1);
LeftLane(2)=A2(1);
LeftLane(3)=A1(1);
LeftLane(4)=A0(1);
LeftLane(5)=Range(1);

%% rightlane

RightLane(1)=A3(2);
RightLane(2)=A2(2);
RightLane(3)=A1(2);
RightLane(4)=A0(2);
RightLane(5)=Range(2);

%% leftre

LeftRe(1)=A3(3);
LeftRe(2)=A2(3);
LeftRe(3)=A1(3);
LeftRe(4)=A0(3);
LeftRe(5)=Range(3);

%% rightre

RightRe(1)=A3(4);
RightRe(2)=A2(4);
RightRe(3)=A1(4);
RightRe(4)=A0(4);
RightRe(5)=Range(4);

== matlab function PvtSubSys_VSM_SCM/LaneAndRe_SignalProcess/InCondition1/VisLineFilter4 ==
  data: EdgeSts output boolean size=4; EdgeA3 output single size=4; EdgeA2 output single; EdgeA1 output single; EdgeA0 output single; tCycle input; VisEdgeSts input size=4; a3 input size=4; a2 input size=4; a1 input size=4; a0 input size=4; R input size=4; LineUpdate input; EdgeUpdate input; dDeltaX input; dDeltaY input; CosOfPsi input; SinOfPsi input; vRef input; EdgeStsK1 input size=4; EdgeA3K1 input size=4; EdgeA2K1 input size=4; EdgeA1K1 input size=4; EdgeA0K1 input size=4; EdgeRangeK1 input; EdgetLostK1 input size=4; EdgeRange output single size=4; EdgetLost output single size=4
function [EdgeSts,EdgeA3,EdgeA2,EdgeA1,EdgeA0,EdgeRange,EdgetLost] = ...
    VisFilter(tCycle,VisEdgeSts,a3,a2,a1,a0,R,LineUpdate,EdgeUpdate,...
    dDeltaX,dDeltaY,CosOfPsi,SinOfPsi,vRef,...
    EdgeStsK1,EdgeA3K1,EdgeA2K1,EdgeA1K1,EdgeA0K1,EdgeRangeK1,EdgetLostK1)

EdgeSts = false(4,1);
EdgeA3 = single(zeros(4,1));
EdgeA2 = single(zeros(4,1));
EdgeA1 = single(zeros(4,1));
EdgeA0 = single(zeros(4,1));
EdgeRange = single(zeros(4,1));
EdgetLost = single(zeros(4,1));

for i=1:2      %Lane
    if (VisEdgeSts(i)>0)&&(LineUpdate==true)  %lanevalid &&lane更新
        EdgeSts(i) = VisEdgeSts(i);
        EdgeA3(i) = a3(i);
        EdgeA2(i) = a2(i);
        EdgeA1(i) = a1(i);
        EdgeA0(i) = a0(i);
        EdgeRange(i) = R(i);
        EdgetLost(i) = single(0);
    else
        EdgetLost(i) = min(EdgetLostK1(i) + tCycle,10); %lane10s内不更新
        if (EdgeStsK1(i)>0)&&(EdgetLost(i)<0.2)   %lanevalid && lost<0.2
            xi = single([0.5*vRef;(0.5*vRef+0.25*EdgeRangeK1(i));(0.5*vRef+0.5*EdgeRangeK1(i));(0.5*vRef+EdgeRangeK1(i))]);
            yi = EdgeA3K1(i)*xi.^3 + EdgeA2K1(i)*xi.^2 + EdgeA1K1(i)*xi + EdgeA0K1(i);
            t_dx = xi-dDeltaX;
            t_dy = yi-dDeltaY;
            TmpX = t_dx*CosOfPsi+t_dy*SinOfPsi;
            TmpY = -t_dx*SinOfPsi+t_dy*CosOfPsi;
            [EdgeA3(i),EdgeA2(i),EdgeA1(i),EdgeA0(i)] = pl(TmpX,TmpY);
            EdgeSts(i) = EdgeStsK1(i);
            EdgeRange(i) = EdgeRangeK1(i) - single(0.25)*vRef*tCycle;
            if EdgeRange(i)<5
               EdgeSts(i) = single(0); 
            end
        else
            EdgeSts(i) = single(0);
            EdgeA3(i) = single(0);
            EdgeA2(i) = single(0);
            EdgeA1(i) = single(0);
            EdgeA0(i) = single(0);
            EdgeRange(i) = single(0);
        end
    end
end
for i=3:4
    if (VisEdgeSts(i)>0)&&(EdgeUpdate==true)
        EdgeSts(i) = VisEdgeSts(i);
        EdgeA3(i) = a3(i);
        EdgeA2(i) = a2(i);
        EdgeA1(i) = a1(i);
        EdgeA0(i) = a0(i);
        EdgeRange(i) = R(i);
        EdgetLost(i) = single(0);
    else
        EdgetLost(i) = min(EdgetLostK1(i) + tCycle,10);
        if (EdgeStsK1(i)>0)&&(EdgetLost(i)<0.2)
            xi =single( [0.5*vRef;(0.5*vRef+0.25*EdgeRangeK1(i));(0.5*vRef+0.5*EdgeRangeK1(i));(0.5*vRef+EdgeRangeK1(i))]);
            yi = EdgeA3K1(i)*xi.^3 + EdgeA2K1(i)*xi.^2 + EdgeA1K1(i)*xi + EdgeA0K1(i);
            t_dx = xi-dDeltaX;
            t_dy = yi-dDeltaY;
            TmpX = t_dx*CosOfPsi+t_dy*SinOfPsi;
            TmpY = -t_dx*SinOfPsi+t_dy*CosOfPsi;
            [EdgeA3(i),EdgeA2(i),EdgeA1(i),EdgeA0(i)] = pl(TmpX,TmpY);
            EdgeSts(i) = EdgeStsK1(i);
            EdgeRange(i) = EdgeRangeK1(i) - single(0.25)*vRef*tCycle;
            if EdgeRange(i)<5
               EdgeSts(i) = single(0);
            end
        else
            EdgeSts(i) =single(0);
            EdgeA3(i) = single(0);
            EdgeA2(i) = single(0);
            EdgeA1(i) = single(0);
            EdgeA0(i) = single(0);
            EdgeRange(i) = single(0);
        end
    end
end

== matlab function PvtSubSys_VSM_SCM/LaneAndRe_SignalProcess/LaneRage_Handle/ELK_laneValid ==
  data: lane1 input; y output single; lane2 input; lane3 input
function y = fcn(lane1,lane2,lane3)
if lane1==single(1)||lane2==single(1)||lane3==single(1)
    y=single(1);
elseif lane1==single(2)||lane2==single(2)||lane3==single(2)
    y=single(2);
else
    y=single(0);
end

== matlab function PvtSubSys_VSM_SCM/LaneAndRe_SignalProcess/LaneRage_Handle/MATLAB Function ==
  data: lane1 input; lane2 input; L output single; lane3 input; L1 input; L2 input
function L= fcn(lane1,lane2,lane3,L1,L2)
if lane2>0&&lane3==single(0)     %有双车道线
    L=L1;
elseif lane2==single(0)&&lane3>0 %两侧存在 车道边界
    L=L2;
elseif lane1>0  %单车道线 或者 无车道线情况
    L=single(3.75);
else          %无车道线情况
    L=single(0);
    
end

== matlab function PvtSubSys_VSM_SCM/LaneAndRe_SignalProcess/LaneRage_Handle/MATLAB Function1 ==
  data: u input; y output single
function y = fcn(u)
y=single(0);
if u<=0.3 && u>0
y = single(1);
end

== matlab function PvtSubSys_VSM_SCM/LaneAndRe_SignalProcess/LaneRage_Handle/MATLAB Function2 ==
  data: u input; y output single
function y = fcn(u)
y=single(0);
if u<=0.3 && u>0
y = single(1);
end

== matlab function PvtSubSys_VSM_SCM/LaneAndRe_SignalProcess/LaneRage_Handle/SameTwoLaneCondition ==
  data: laneleft_valid input; laneright_valid input; releft_valid input; reright_valid input; laneleft input; laneright input; releft input; reright input; L1 output single; lane output single
function [L1, lane] =fcn(laneleft_valid,laneright_valid,releft_valid,reright_valid,...
    laneleft,laneright,releft,reright)

if laneleft_valid==single(1)&&laneright_valid==single(1)&&releft_valid==single(0)&&reright_valid==single(0)&&laneleft<laneright
    lane=single(1); %access lane_left
    L1=laneleft+laneright;
elseif laneleft_valid==single(1)&&laneright_valid==single(1)&&releft_valid==single(0)&&reright_valid==single(0)&&laneleft>laneright
    lane=single(2);
    L1=laneleft+laneright;
elseif laneleft_valid==single(0)&&laneright_valid==single(0)&&releft_valid==single(1)&&reright_valid==1&&releft<reright
    lane=single(3); %access re_left
    L1=releft+reright;
elseif laneleft_valid==single(0)&&laneright_valid==single(0)&&releft_valid==single(1)&&reright_valid==single(1)&&releft>reright
    lane=single(4);
    L1=releft+reright;

else
    lane=single(0);
    L1=single(0);
    
end

== matlab function PvtSubSys_VSM_SCM/LaneAndRe_SignalProcess/LaneRage_Handle/SingleLaneCondition ==
  data: laneleft_valid input; lane output single; laneright_valid input; releft_valid input; reright_valid input
function lane = fcn(laneleft_valid,laneright_valid,releft_valid,reright_valid)
if laneleft_valid==single(1)&&laneright_valid==single(0)&&releft_valid==single(0)&&reright_valid==single(0)
    lane=single(1);%lane=1 左侧车道线（判断条件是 只有左侧车道线 ）
elseif laneleft_valid==single(0)&&laneright_valid==single(1)&&releft_valid==single(0)&&reright_valid==single(0)
    lane=single(2);
elseif laneleft_valid==single(0)&&laneright_valid==single(0)&&releft_valid==single(1)&&reright_valid==single(0)
    lane=single(3);
elseif laneleft_valid==single(0)&&laneright_valid==single(0)&&releft_valid==single(0)&&reright_valid==single(1)
    lane=single(4);
else
    lane=single(0);
end

== matlab function PvtSubSys_VSM_SCM/LaneAndRe_SignalProcess/LaneRage_Handle/Subsystem/MATLAB Function3 ==
  data: Left_a0 input; T_A0 output single; Left_a1 input; T_A1 output single; T_A2 output single; T_A3 output single; T_Range output single; T_Valid output boolean; C_Lanewidth output single; Left_a2 input; Left_a3 input; Left_range input; Left_Valid input; Right_a0 input; Right_a1 input; Right_a2 input; Right_a3 input; Right_range input; Right_Valid input; Center_a0 input; Center_a1 input; Center_a2 input; Center_a3 input; Center_valid input; LKAOffset input
function [T_A0,T_A1,T_A2,T_A3,T_Range,T_Valid,C_Lanewidth] = fcn(Left_a0,Left_a1,Left_a2,Left_a3,Left_range,Left_Valid,......
    Right_a0,Right_a1,Right_a2,Right_a3,Right_range,Right_Valid,Center_a0,Center_a1,Center_a2,Center_a3,Center_valid,LKAOffset)


C_Lanewidth=Left_a0 - Right_a0;
if Center_valid>0
    T_A0=Center_a0;
    T_A1=Center_a1;
    T_A2=Center_a2;
    T_A3=Center_a3;
    T_Range=max(Left_range ,Right_range);
    T_Valid=Center_valid;
elseif Left_Valid>0 && Right_Valid>0 && (Left_a0 - Right_a0)<5.5
    T_A0=(Left_a0 + Right_a0)/2;
    T_A1=(Left_a1 + Right_a1)/2;
    T_A2=(Left_a2 + Right_a2)/2;
    T_A3=(Left_a3 + Right_a3)/2;
    T_Range=max(Left_range ,Right_range);
    T_Valid=true;
elseif Left_Valid>0 && Right_Valid>0 && (Left_a0 - Right_a0)>=5.5
    if abs(Left_a0)-abs(Right_a0)>0
        T_A0=Right_a0+LKAOffset;
        T_A1=Right_a1;
        T_A2=Right_a2;
        T_A3=Right_a3;
        T_Range=Right_range;
        T_Valid=Right_Valid;
        C_Lanewidth=single(3.75);
    else
        T_A0=Left_a0-LKAOffset;
        T_A1=Left_a1;
        T_A2=Left_a2;
        T_A3=Left_a3;
        T_Range=Left_range;
        T_Valid=Left_Valid;
        C_Lanewidth=single(3.75);
    end
elseif Left_Valid>0 && Right_Valid==0
    T_A0=Left_a0-LKAOffset;
    T_A1=Left_a1;
    T_A2=Left_a2;
    T_A3=Left_a3;
    T_Range=Left_range;
    T_Valid=Left_Valid;
    C_Lanewidth=single(3.75);
elseif  Left_Valid==0 && Right_Valid>0
    T_A0=Right_a0+LKAOffset;
    T_A1=Right_a1;
    T_A2=Right_a2;
    T_A3=Right_a3;
    T_Range=Right_range;
    T_Valid=Right_Valid;
    C_Lanewidth=single(3.75);
else
    T_A0=single(0);
    T_A1=single(0);
    T_A2=single(0);
    T_A3=single(0);
    T_Range=single(0);
    T_Valid=false;
    C_Lanewidth=single(0);
end

== matlab function PvtSubSys_VSM_SCM/LaneAndRe_SignalProcess/LaneRage_Handle/TwoLaneCondition ==
  data: laneleft_valid input; lane output single; laneright_valid input; releft_valid input; reright_valid input; laneleft input; laneright input; releft input; reright input; L2 output single
function [lane,L2] =fcn(laneleft_valid,laneright_valid,releft_valid,reright_valid,...
    laneleft,laneright,releft,reright)
%线与边界
if laneleft_valid==single(1)&&laneright_valid==single(0)&&releft_valid==single(0)&&reright_valid==single(1)&&laneleft<reright
    lane=single(1); % access lane_left
    L2=laneleft+reright;
elseif laneleft_valid==single(1)&&laneright_valid==single(0)&&releft_valid==single(0)&&reright_valid==single(1)&&laneleft>reright
    lane=single(4);
    L2=laneleft+reright;
elseif laneleft_valid==single(0)&&laneright_valid==single(1)&&releft_valid==single(1)&&reright_valid==single(0)&&laneright<releft
    lane=single(2); % access lane_right
    L2=laneright+releft;
elseif laneleft_valid==single(0)&&laneright_valid==single(1)&&releft_valid==single(1)&&reright_valid==single(0)&&laneright>releft
    lane=single(3);
    L2=laneright+releft;

else
    lane=single(0);
    L2=single(0);
end

== matlab function PvtSubSys_VSM_SCM/LaneAndRe_SignalProcess/LaneRage_Handle/CalcEgoVehMove1 ==
  data: dDeltaX output single size=1; tCycle input single size=1; Kap input single size=1; Vego input single size=1; dDeltaY output single size=1; CosOfPsi output single size=1; SinOfPsi output single size=1
function [dDeltaX,dDeltaY,CosOfPsi,SinOfPsi] = EgoVehicleMovement(tCycle,Kap,Vego)
%#codegen
if Kap==0
    dDeltaX = Vego*tCycle;
    dDeltaY = single(0);
    CosOfPsi = single(1);
    SinOfPsi = single(0);
else
    t_Psi = Kap*Vego*tCycle;
    SinOfPsi = sin(t_Psi);
    CosOfPsi = cos(t_Psi);
    dDeltaX = SinOfPsi/Kap;
    dDeltaY = 2*(sin(t_Psi/2)*sin(t_Psi/2))/Kap;
end

== matlab function PvtSubSys_VSM_SCM/LaneAndRe_SignalProcess/LaneRage_Handle/Tracker ==
  data: LeftOffset_b output boolean size=1; RightOffset_b output boolean size=1; LineUpdate input boolean size=1; LineConf input uint8 size=2; A0 input single size=2; A1 input single size=2; A2 input single size=2; A3 input single size=2; dDeltaX input single size=1; dDeltaY input single size=1; CosOfPsi input single size=1; SinOfPsi input single size=1; vRef input single size=1; error_right output single size=1; error_left output single size=1; pre_A1_2 output single size=1; pre_A0_2 output single size=1; pre_A1_1 output single size=1; pre_A0_1 output single size=1; pre_A1_2K1 input single size=1; pre_A0_2K1 input single size=1; pre_A1_1K1 input single size=1; pre_A0_1K1 input single size=1; pre_LineConfK1 input uint8 size=2; pre_LineConf output uint8 size=2
function [LeftOffset_b,RightOffset_b,error_right,error_left,pre_A1_2,pre_A0_2,...
    pre_A1_1,pre_A0_1,pre_LineConf] = ...
    LineTracker(LineUpdate,LineConf,A0,A1,A2,A3,...
    dDeltaX,dDeltaY,CosOfPsi,SinOfPsi,vRef,pre_A1_2K1,pre_A0_2K1,...
    pre_A1_1K1,pre_A0_1K1,pre_LineConfK1)

LeftOffset_b = false;
RightOffset_b = false;
error_right = single(3.5);
error_left = single(3.5);
pre_LineConf = LineConf;
t_Dist = max(single(15),vRef*1.8);
x = [0.05*t_Dist;0.3*t_Dist;0.6*t_Dist;t_Dist];
y2 = A3(2)*x.^3 + A2(2)*x.^2 + A1(2)*x + A0(2);%右侧
y1 = A3(1)*x.^3 + A2(1)*x.^2 + A1(1)*x + A0(1);%左侧
t_dx = x-dDeltaX;
t_dy2 = y2-dDeltaY;
t_dy1 = y1-dDeltaY;
TmpX2 = t_dx*CosOfPsi+t_dy2*SinOfPsi;
TmpY2 = -t_dx*SinOfPsi+t_dy2*CosOfPsi;
TmpX1 = t_dx*CosOfPsi+t_dy1*SinOfPsi;
TmpY1 = -t_dx*SinOfPsi+t_dy1*CosOfPsi;
[pre_A3_2,pre_A2_2,pre_A1_2,pre_A0_2] = pl(TmpX2,TmpY2);
[pre_A3_1,pre_A2_1,pre_A1_1,pre_A0_1] = pl(TmpX1,TmpY1);
if LineUpdate
    error_right = abs(A0(2)-pre_A0_1K1);
    error_left = abs(A0(1)-pre_A0_2K1);
    if error_right<0.7 && pre_LineConfK1(1)>0 && LineConf(1)>0 && abs(57.3*(atan(A1(1))-atan(pre_A1_1K1)))<5
        LeftOffset_b = false;
        RightOffset_b = true;
    elseif error_left<0.7 && pre_LineConfK1(2)>0 && LineConf(2)>0 && abs(57.3*(atan(A1(2))-atan(pre_A1_2K1)))<5
        LeftOffset_b = true;
        RightOffset_b = false;
    end
end
% if LineUpdate
%     error_right = abs(A0(1)-pre_A0_1K1);
%     error_left = abs(A0(3)-pre_A0_2K1);
%     if error_right<0.7 && pre_LineConfK1(3)>0 && LineConf(2)>0 && abs(57.3*(atan(A1(2))-atan(pre_A1_3K1)))<5
%         LeftOffset_b = false;
%         RightOffset_b = true;
%     elseif error_left<0.7 && pre_LineConfK1(2)>0 && LineConf(3)>0 && abs(57.3*(atan(A1(3))-atan(pre_A1_2K1)))<5
%         LeftOffset_b = true;
%         RightOffset_b = false;
%     end
% end
